simulink model "Part2_Peregrine_Falcon_Dive"  (R2022b)
settings: Solver=VariableStepAuto  StartTime=0.0  StopTime=10.0  RelTol=1e-3
undefined symbols (not defined in the file): A1, A2, Cd1, Cd2, g, m, rho
settings Model: Creator=Haina Bhawnani  LastModifiedBy=Haina Bhawnani

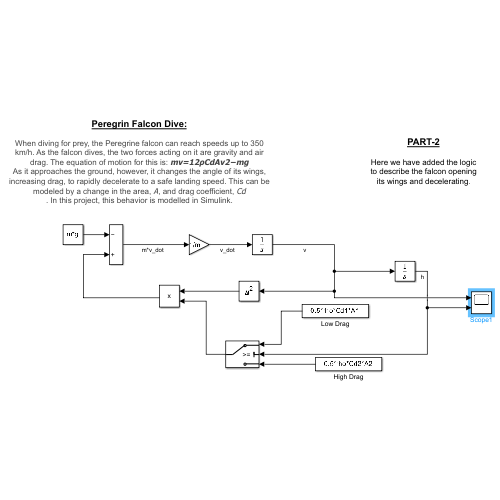
[thumbnail: Simulink's stored preview of the top-level diagram]
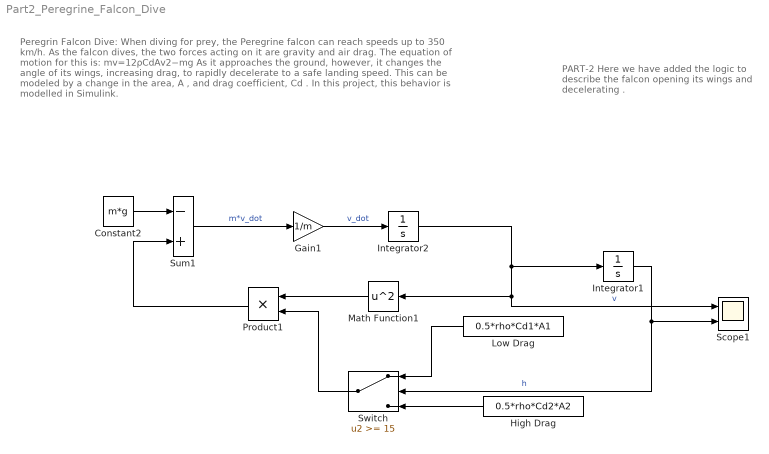
== system Part2_Peregrine_Falcon_Dive ==
  note: PART-2
      |
      | Here we have added the logic to describe the falcon opening its wings and decelerating .
  note: Peregrin Falcon Dive:
      |
      | When diving for prey, the Peregrine falcon can reach speeds up to 350 km/h. As the falcon dives, the two forces acting on it are gravity and air drag. The equation of motion for this is: mv=12ρCdAv2−mg
      | As it approaches the ground, however, it changes the angle of its wings, increasing drag, to rapidly decelerate to a safe landing speed. This can be modeled by a change in the area, A , and drag coefficient, Cd
      | . In this project, this behavior is modelled in Simulink.
  Constant2 : Constant  Value=m*g
  Gain1 : Gain  Gain=1/m
  High Drag : Constant  Value=0.5*rho*Cd2*A2
  Integrator1 : Integrator  InitialCondition=60
  Integrator2 : Integrator  InitialCondition=-10
  Low Drag : Constant  Value=0.5*rho*Cd1*A1
  Math Function1 : Math  Operator=square  SignedPower=on
  Product1 : Product
  Scope1 : Scope  NumInputPorts=2
  Sum1 : Sum  Inputs=-+
  Switch : Switch  Threshold=15  SaturateOnIntegerOverflow=off  InputSameDT=off
  wires:
  Integrator1/1 -> Scope1/2, Switch/2  "h"
  Switch/1 -> Product1/2
  Math Function1/1 -> Product1/1
  Integrator2/1 -> Scope1/1, Math Function1/1, Integrator1/1  "v"
  Constant2/1 -> Sum1/1
  Product1/1 -> Sum1/2
  Sum1/1 -> Gain1/1  "m*v_dot"
  Low Drag/1 -> Switch/1
  Gain1/1 -> Integrator2/1  "v_dot"
  High Drag/1 -> Switch/3
